simulink model "Force_control_compliance_3link"  (R2020b)
settings: Solver=VariableStepAuto  StartTime=0.0  StopTime=10.0  RelTol=1e-3
InitFcn:
  | wks = get_param('f','ModelWorkspace');
  | reload(wks)
model workspace: external: MAT-File C:\Users\Anna Rothweil\Documents\MAE547\Final Report\3-Link\globals.mat (data not in the file)
values from neighbouring files (symbols this model uses):
  dh_calc = dh_syms(:)    [compliance_control.m]    (also in compliance_control_3link.m = double(dh_syms))
  Fneg = Fc(:,2)-Fb    [EOMFinder.m]
  Fpos = Fc(:,1)+Fb    [EOMFinder.m]
  he = eval(subs(heFunc,t,time))    [complianceControl.m]    (also in impedanceControl.m)
  J = Arm.jacob0(q.')    [JFinder.m]
undefined symbols (not defined in the file or in its folder): FB
settings Model: Creator=Anna Rothweil  LastModifiedBy=Anna Rothweil
settings DebuggingCC: UnderSpecifiedDimensionMsg=warning
settings SFSimCC: MATLABDynamicMemAllocThreshold=0  CustomCodeUndefinedFunction=UseInterfaceOnly

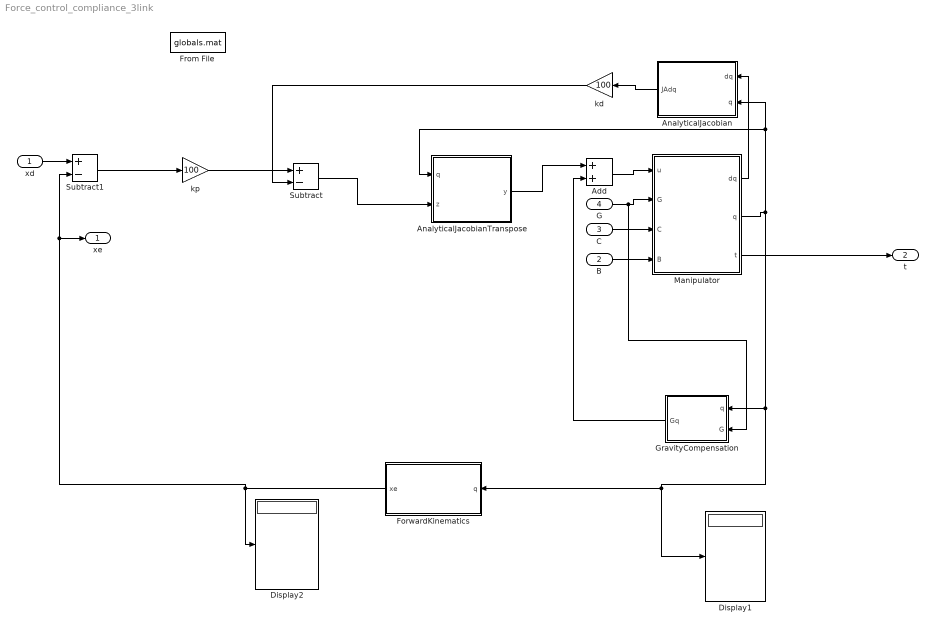
== system Force_control_compliance_3link ==
  xd : Inport  PortDimensions=6  SampleTime=0.01
  B : Inport  Port=2  SampleTime=0.01
  C : Inport  Port=3  SampleTime=0.01
  G : Inport  Port=4  SampleTime=0.01
  Add : Sum
  AnalyticalJacobian : MATLAB Function  TreatAsAtomicUnit=on
  AnalyticalJacobianTranspose : MATLAB Function  TreatAsAtomicUnit=on
  Display1 : Display
  Display2 : Display
  ForwardKinematics : MATLAB Function  TreatAsAtomicUnit=on
  From File : FromFile  FileName=globals.mat  SampleTime=0.01
  GravityCompensation : MATLAB Function  TreatAsAtomicUnit=on
  Manipulator : Subsystem
  Subtract : Sum  Inputs=+-
  Subtract1 : Sum  Inputs=+-
  kd : Gain  Gain=100
  "kp " : Gain  Gain=100
  xe : Outport  PortDimensions=[6,1]  SampleTime=0.01
  t : Outport  Port=2
  wires:
  Subtract1/1 -> "kp "/1
  GravityCompensation/1(Gq) -> Add/2
  Subtract/1 -> AnalyticalJacobianTranspose/2(z)
  AnalyticalJacobianTranspose/1(y) -> Add/1
  kd/1 -> Subtract/2
  "kp "/1 -> Subtract/1
  xd/1 -> Subtract1/1
  Manipulator/1(dq) -> AnalyticalJacobian/1(dq)
  Manipulator/2("q ") -> AnalyticalJacobianTranspose/1(q), AnalyticalJacobian/2(q), Display1/1, ForwardKinematics/1(q), GravityCompensation/1(q)
  Add/1 -> Manipulator/1(u)
  ForwardKinematics/1(xe) -> xe/1, Subtract1/2, Display2/1
  B/1 -> Manipulator/4(B)
  C/1 -> Manipulator/3(C)
  G/1 -> GravityCompensation/2(G), Manipulator/2(G)
  AnalyticalJacobian/1(JAdq) -> kd/1
  Manipulator/3(t) -> t/1

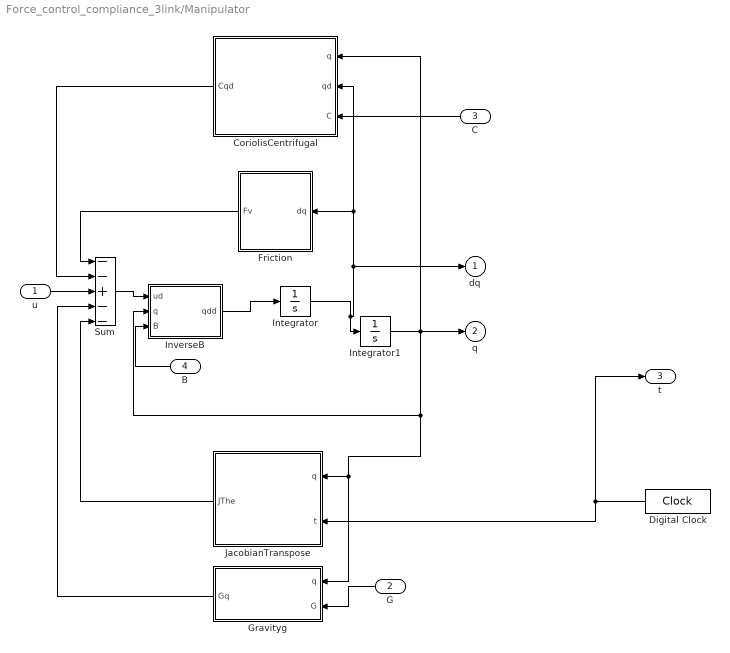
== system Force_control_compliance_3link/Manipulator ==
  u : Inport  SampleTime=0.01
  G : Inport  Port=2  SampleTime=0.01
  C : Inport  Port=3
  B : Inport  Port=4
  CoriolisCentrifugal : MATLAB Function  TreatAsAtomicUnit=on
  Digital Clock : DigitalClock  SampleTime=0.01
  Friction : MATLAB Function  TreatAsAtomicUnit=on
  Gravityg : MATLAB Function  TreatAsAtomicUnit=on
  Integrator : Integrator  InitialCondition=[0;0;0]
  Integrator1 : Integrator  InitialCondition=[0;0;0]
  InverseB : MATLAB Function  TreatAsAtomicUnit=on
  JacobianTranspose : MATLAB Function  TreatAsAtomicUnit=on
  Sum : Sum  Inputs=--+--  InputSameDT=on  SaturateOnIntegerOverflow=on  OutDataTypeStr=Inherit: Same as first input
  dq : Outport  SampleTime=0.01  InitialOutput=0
  "q " : Outport  Port=2  SampleTime=0.01  InitialOutput=0
  t : Outport  Port=3
  wires:
  InverseB/1(qdd) -> Integrator/1
  Integrator/1 -> Integrator1/1, dq/1, CoriolisCentrifugal/2(qd), Friction/1(dq)
  CoriolisCentrifugal/1(Cqd) -> Sum/2
  Friction/1(Fv) -> Sum/1
  u/1 -> Sum/3
  Integrator1/1 -> Gravityg/1(q), JacobianTranspose/1(q), InverseB/2(q), CoriolisCentrifugal/1(q), "q "/1
  Gravityg/1(Gq) -> Sum/4
  JacobianTranspose/1(JThe) -> Sum/5
  Sum/1 -> InverseB/1(ud)
  Digital Clock/1 -> t/1, JacobianTranspose/2(t)
  G/1 -> Gravityg/2(G)
  C/1 -> CoriolisCentrifugal/3(C)
  B/1 -> InverseB/3(B)

== matlab function Force_control_compliance_3link/Manipulator/CoriolisCentrifugal ==
  data: q input size=[3,1]; Cqd output size=[3,1]; qd input size=[3,1]; C input size=[3,3]
function Cqd = fcn(q, qd, C)
n=3;
coder.extrinsic('CFinder');
Cq = zeros(n,n);
Cq = CFinder(C, q, qd);
Cqd=zeros(n,1);
Cqd=Cq*qd;
%coder.varsize('Cqd', [20,1], [1 0]);
end

== matlab function Force_control_compliance_3link/AnalyticalJacobianTranspose ==
  data: q input size=[3,1]; z input size=[6,1]; y output size=[3,1]; dh_calc parameter size=[12,1]; J parameter size=[3,1]
function y = fcn(q, z, dh_calc, J)
%dh_calc: the 4*N x 1 vector of symbolic dh parameters (numbers)
%convert dh_calc to matrix form of size Nx4
%n=size(dh_calc,1);
%assert (n <= 20);
n=3;
dh_calc2 = zeros(n,4);
w=1;
for j=1:4
    for i=1:n
        dh_calc2(i,j) = dh_calc(w);
        w=w+1;
    end
end

%z must be 6x1
coder.extrinsic('JAFinder');
JA=zeros(6,n);
JA = JAFinder(dh_calc2, q, J);
y=zeros(n,1);
y=JA.'*z;
%coder.varsize('y', [20,1], [1 0]);
end

== matlab function Force_control_compliance_3link/ForwardKinematics ==
  data: q input size=[3,1]; xe output size=[6,1]; dh_calc parameter size=[12,1]; J parameter size=[3,1]
function xe = fcn(q, dh_calc, J)

%dh_calc; size Nx4, numeric DH parameters
n=3;
%q: Nx1 matrix of joint parameters
%T: 4x4 homogeneous transformation matrix

%I think this code is not working because Arm is symbolic
%let's evaluate Arm first before using it with fkine
coder.extrinsic('ArmFinder');
xe=zeros(6,1);
xe=ArmFinder(dh_calc,q,J);

% s=size(xe,1)
% if s==6
%     xe=xe;
% else
%     xe=zeros(6,1)
%     fprintf('xe is zeros - FWD KIN error')
end

== matlab function Force_control_compliance_3link/Manipulator/Gravityg ==
  data: q input size=[3,1]; Gq output size=[3,1]; G input size=[3,1]
function Gq = fcn(q, G)
n=3;
coder.extrinsic('GFinder');
%n=size(G, 1);
%assert (n <= 20);
Gq = zeros(n,1);
%coder.varsize('Gq', [20,1], [1 0]);
Gq = GFinder(G, q);
end

== matlab function Force_control_compliance_3link/AnalyticalJacobian ==
  data: dq input size=[3,1]; JAdq output size=[6,1]; q input size=[3,1]; dh_calc parameter size=[12,1]; J parameter size=[3,1]
function JAdq = fcn(dq, q, dh_calc, J)
%dh_calc: the N x 4 vector of dh parameters (numbers)
n=3;
%n=size(dh_calc,1);
%assert (n <= 20);

coder.extrinsic('JAFinder');
JA=zeros(6,n);
JA = JAFinder(dh_calc, q, J);
JAdq=zeros(6,1);
JAdq=JA*dq;
end

== matlab function Force_control_compliance_3link/GravityCompensation ==
  data: q input size=[3,1]; Gq output size=[3,1]; G input size=[3,1]
function Gq = fcn(q, G)
%n=size(Gq,1);
%assert (n <= 20);
n=3;
coder.extrinsic('GFinder');
Gq = zeros(n,1);
Gq= GFinder(G, q);
%coder.varsize('Gq', [20,1], [1 0]);
end

== matlab function Force_control_compliance_3link/Manipulator/JacobianTranspose ==
  data: q input size=[3,1]; JThe output size=[3,1]; t input size=1; he parameter size=[6,1]; J parameter size=[3,1]; dh_calc parameter size=[12,1]
function JThe = fcn(q, t, he, J, dh_calc)
%dh_calc: nx4
n=3;

coder.extrinsic('JFinder');
Jg=zeros(6,n);
he_calc=zeros(6,1);
[Jg, he_calc] = JFinder(dh_calc, q, J, he, t);

JThe=zeros(n,1);
JThe=(Jg.')*he_calc;
%coder.varsize('JThe', [20,1], [1 0]);
end

== matlab function Force_control_compliance_3link/Manipulator/Friction ==
  data: dq input size=[3,1]; Fv output size=[3,1]; FB parameter size=[3,1]; Fpos parameter size=[3,1]; Fneg parameter size=[3,1]
function Fv = fcn(dq, FB, Fpos, Fneg)
%F is friction is  NxN
%Fv is F*dq and is Nx1
%n=size(FB,1);
%assert (n <= 20);
%create vector of friction coefficients
%n=3;
Fv=zeros(3,1);
for i=1:3
    if dq(i)>0
        Fv(i)= FB(i)*dq(i)+Fpos(i);
    else if dq(i)<0
        Fv(i)= FB(i)*dq(i)+Fneg(i);
    else
        Fv(i)=0;
    end
    end

%coder.varsize('Fv', [3,1], [1 0]);
end

== matlab function Force_control_compliance_3link/Manipulator/InverseB ==
  data: ud input size=[3,1]; q input size=[3,1]; qdd output size=[3,1]; B input size=[3,3]
function qdd = fcn(ud,q, B)
%ud and q must be Nx1
%B is NxN
n=3;
coder.extrinsic('BFinder');
Bq = zeros(n,n);
Bq = BFinder(B, q);
%Binv is also NxN
Binv=inv(Bq);
%qdd must be nx1
qdd=zeros(n,1);
qdd=Binv*ud;
%coder.varsize('qdd', [20,1], [1 0]);
